simulink model "Torque_Vectoring_Controller_dSpace_RTI1401"  (R2016a)
settings: Solver=ode1  StartTime=0.0  StopTime=Inf  FixedStep=car.dt  RelTol=1e-3
PostLoadFcn:
  | , if any(exist('dsrtsu_mdlpostloadfcn', 'file') == [2, 3, 6]), try dsrtsu_mdlpostloadfcn('Execute', bdroot); catch fprintf('Error in PostLoadFcn (dsrtsu_mdlpostloadfcn) for model "%s":\n %s\n', bdroot, lasterr); end, end,
InitFcn:
  | clear_close
  | dataCar
  | optParam
  | structSensors
  | structSettings
  | structEstimPar
  | structAero
  | structVariables
  | readFuzzyFile
StartFcn:
  | clear_close
  | dataCar
  | optParam
  | structSensors
  | structSettings
  | structEstimPar
  | structAero
  | structVariables
  | readFuzzyFile
undefined symbols (not defined in the file or in its folder): car, optPar
libraries: fuzblock x1
(part 1 of 2)
PreSaveFcn:
  | , if any(exist('dsmpb_private', 'file') == [2, 3, 6]), try, dsmpb_private('dsmpb_mdlclblib', 'PreSave', bdroot); catch, disp(lasterr); end, end,
CloseFcn:
  | , if any(exist('dsmpb_private', 'file') == [2, 3, 6]), try, dsmpb_private('dsmpb_mdlclblib', 'Close', bdroot); catch, disp(lasterr); end, end,
settings Model: DSRTSU_INTERNAL_RTI_VER=490  DSRTSU_INTERNAL_RTI_TYPE=rti1401  DSRTSU_INTERNAL_RTIFPGA=80  DSMPB_DATASERVER_ModelPortLibVersion1=8  DSMPB_DATASERVER_DataServerVersion1=6  DSMPB_DATASERVER_DataServerStreamVersion1=3  Creator=Boon  LastModifiedBy=Boon
settings OptimizationCC: BlockReduction=off  OptimizeBlockIOStorage=off  BufferReuse=off  GlobalBufferReuse=off  ExpressionFolding=off  LocalBlockOutputs=off
settings HardwareCC: ProdBitPerPointer=32  ProdLargestAtomicInteger=Integer  ProdEndianess=BigEndian  ProdWordSize=32  ProdHWDeviceType=Custom Processor->Custom  TargetIntDivRoundTo=Zero  TargetEndianess=BigEndian  TargetHWDeviceType=Custom Processor->Custom
settings RTWCC: SystemTargetFile=rti1401.tlc  MakeCommand=make_rti  TemplateMakefile=rti1401.tmf  Description=dSPACE DS1401 Hardware Platform
settings STFCustomTargetCC: ParMdlRefBuildCompliant=on  GRTInterface=off  SystemTargetFile=rti1401.tlc
settings GRTTargetCC: CompOptLevelCompliant=off  ConcurrentExecutionCompliant=off  GeneratePreprocessorConditionals=Use local settings  CombineOutputUpdateFcns=off  MatFileLogging=off  CPPClassGenCompliant=off  UseToolchainInfoCompliant=off

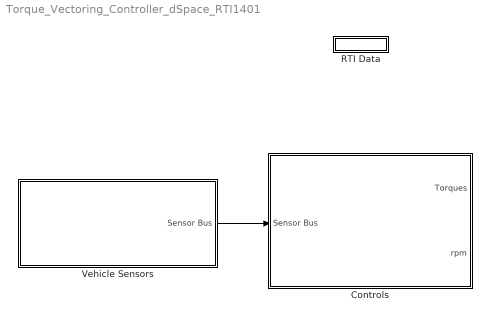
== system Torque_Vectoring_Controller_dSpace_RTI1401 ==
  Controls : Subsystem
  RTI Data : Subsystem  Tag=struct('RTIDataServer',struct('RTIDataServerVs','2','RTIModelDescription','struct(''main'',''Torque_Vectoring_Controller_dSpace_RTI1401'',''sub'','''',''isMp'',0)'))  LoadFcn="if exist('rtidc'), try,  rtidc('DataHostBlockClbLoad', gcbh); catch, disp(['Warning: ''LoadFcn'' for RTI Data block failed: ' lasterr]); end, end,"  mask(RTI_DATA_HOST){}
      mask help:
      | RTI Data Block.
      | This block is used by RTI to store internal model-dependent data.
      | Please keep this block on the root level of the model. Deleting this block will result in data loss.
      |
      | NEVER DELETE OR COPY THIS BLOCK!
      settings: CopyFcn="if exist('rtidc'), try,  rtidc('DataHostBlockClbCopy', gcbh); catch, disp(['Warning: ''CopyFcn'' for RTI Data block failed: ' lasterr]); end, end,"  DeleteFcn="if exist('rtidc'), try,  rtidc('DataHostBlockClbDelete', gcbh); catch, disp(['Warning: ''DeleteFcn'' for RTI Data block failed: ' lasterr]); end, end,"  ModelCloseFcn="if exist('rtidc'), try,  rtidc('DataHostBlockClbModelClose', gcbh); catch, disp(['Warning: ''ModelCloseFcn'' for RTI Data block failed: ' lasterr]); end, end,"  PreSaveFcn="if exist('rtidc'), try,  rtidc('DataHostBlockClbPreSave', gcbh); catch, disp(['Warning: ''PreSaveFcn'' for RTI Data block failed: ' lasterr]); end, end,"  PostSaveFcn="if exist('rtidc'), try,  rtidc('DataHostBlockClbPostSave', gcbh); catch, disp(['Warning: ''PostSaveFcn'' for RTI Data block failed: ' lasterr]); end, end,"  NameChangeFcn="if exist('rtidc'), try,  rtidc('DataHostBlockClbNameChange', gcbh); catch, disp(['Warning: ''NameChangeFcn'' for RTI Data block failed: ' lasterr]); end, end,"
      mask Help:
      | RTI Data Block.
      | This block is used by RTI to store internal model-dependent data.
      | Please keep this block on the root level of the model. Deleting this block will result in data loss.
      | 
      | NEVER DELETE OR COPY THIS BLOCK!
      mask Display:
      | text(0.5, 0.5, 'RTI Data', 'HorizontalAlignment', 'center');
      | plot([1 0]);
  Vehicle Sensors : Subsystem
  wires:
  Vehicle Sensors/1(" Sensor Bus") -> Controls/1(Sensor Bus)

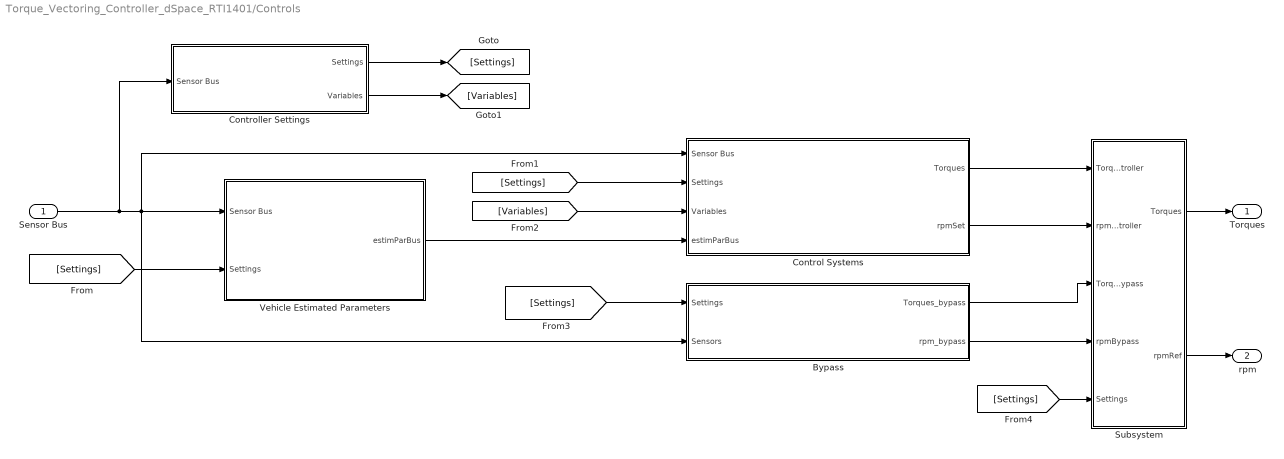
== system Torque_Vectoring_Controller_dSpace_RTI1401/Controls ==
  Sensor Bus : Inport
  Bypass : Subsystem
  Control Systems : Subsystem
  Controller Settings : Subsystem
  Subsystem : Subsystem
  Vehicle Estimated Parameters : Subsystem
  Torques : Outport
  rpm : Outport  Port=2
  wires:
  Sensor Bus/1 -> Controller Settings/1(Sensor Bus), Bypass/2(Sensors), Control Systems/1(Sensor Bus), Vehicle Estimated Parameters/1(Sensor Bus)
  [Settings] -> Vehicle Estimated Parameters/2(Settings)
  Vehicle Estimated Parameters/1(" estimParBus") -> Control Systems/4(estimParBus)
  Controller Settings/1(Settings) -> [Settings]
  [Settings] -> Control Systems/2(Settings)
  Controller Settings/2(Variables) -> [Variables]
  [Variables] -> Control Systems/3("Variables ")
  [Settings] -> Bypass/1(Settings)
  Control Systems/1(Torques) -> Subsystem/1(TorqueController)
  Subsystem/1(Torques) -> Torques/1
  Bypass/2(rpm_bypass) -> Subsystem/4(rpmBypass)
  Bypass/1(Torques_bypass) -> Subsystem/3(TorqueBypass)
  [Settings] -> Subsystem/5(Settings)
  Control Systems/2(rpmSet) -> Subsystem/2(rpmController)
  Subsystem/2(rpmRef) -> rpm/1

== system Torque_Vectoring_Controller_dSpace_RTI1401/RTI Data ==
  RTI Data Store : Subsystem  Tag="struct('private',struct('version',struct('dsVer',uint32(2),'dsVerCreation',uint32(2),'RTI',struct('ver','7.7','type','RTI1401')),'access',struct('type','Model','isPerm',1,'created',['18-Apr-2017 22:43:45'],'modified',['26-Apr-2017 00:23:53'],'location','')),'public',struct('main',struct('data',[]),'sub',struct('name',{{'Torque_Vectoring_Controller_dSpace_RTI1401'}},'data',{{struct('TH',struct('thTaskInfo',struct('taskType',{'TIMER','HWINT','TMRINT','SWINT','GLINT'},'tasksNumOf',{1,0,0,0,0},'srcIds',{{'TIMERA'},{},{},{},{}},'taskNames',{{['Timer Task 1']},{},{},{},{}})),'th_tc',struct('dataType','TASK','taskGroupId','','taskGroupList',{{}},'taskSchedulingPolicy','FCFS','taskType','TIMER','blkh',-1,'srcId','TIMERA','srcSgnName',['Timer A interrupt'],'srcCpuName','','taskName',['Timer Task 1  [0.001] s'],'taskNameDisplayExt','','smplTime',0.001,'smplTimeOffs',0,'hasFixedPriority',0,'priority',1,'hasFixedOvc',0,'ovcType',1,'ovcMax',1),'tc_th',struct('dataType','TASK','taskGroupId','','taskGroupList',{{}},'taskSchedulingPolicy','FCFS','taskType','TIMER','blkh',-1,'srcId','TIMERA','srcSgnName',['Timer A interrupt'],'srcCpuName','','taskName',['Timer Task 1  [0.001] s'],'taskNameDisplayExt','','smplTime',0.001,'smplTimeOffs',0,'hasFixedPriority',0,'priority',1,'hasFixedOvc',0,'ovcType',1,'ovcMax',1))}})))"  mask(RTI_DATA_STORE){}
      mask help:
      | RTI Data Store Block. This block is used by RTI to store internal model dependent data. Deleting this block will result in data loss.
      |
      | NEVER DELETE, COPY, OR MODIFY THIS BLOCK!
      mask Help:
      | RTI Data Store Block. This block is used by RTI to store internal model dependent data. Deleting this block will result in data loss.
      | 
      | NEVER DELETE, COPY, OR MODIFY THIS BLOCK!
      mask Display: text(0.5, 0.5, ' ', 'HorizontalAlignment', 'center');

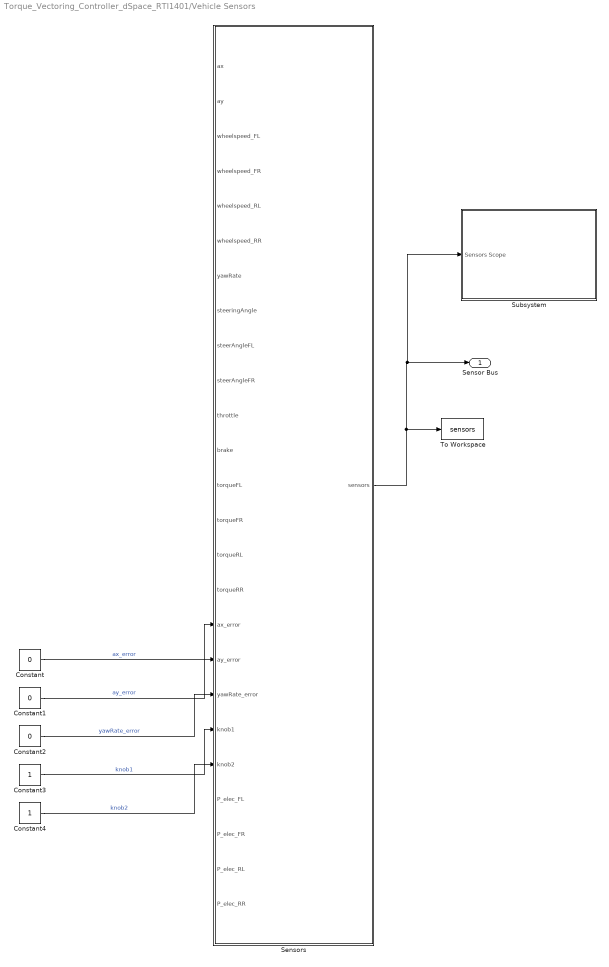
== system Torque_Vectoring_Controller_dSpace_RTI1401/Vehicle Sensors ==
  Constant : Constant  Value=0
  Constant1 : Constant  Value=0
  Constant2 : Constant  Value=0
  Constant3 : Constant
  Constant4 : Constant
  Sensors : MATLAB Function  TreatAsAtomicUnit=on
  Subsystem : Subsystem
      mask Display: image('Sensors Scope.png');
  To Workspace : ToWorkspace  VariableName=sensors  SaveFormat=Timeseries  SampleTime=-1
  " Sensor Bus" : Outport
  wires:
  Constant4/1 -> Sensors/21(knob2)  "knob2"
  Constant3/1 -> Sensors/20(knob1)  "knob1"
  Constant2/1 -> Sensors/19(yawRate_error)  "yawRate_error"
  Constant1/1 -> Sensors/18(ay_error)  "ay_error"
  Constant/1 -> Sensors/17(ax_error)  "ax_error"
  Sensors/1(sensors) -> Subsystem/1("Sensors Scope "), " Sensor Bus"/1, To Workspace/1

== system Torque_Vectoring_Controller_dSpace_RTI1401/Controls/Bypass ==
  Settings : Inport
  Sensors : Inport  Port=2
  MATLAB Function : MATLAB Function  TreatAsAtomicUnit=on
  Torques_bypass : Outport
  rpm_bypass : Outport  Port=2
  wires:
  Settings/1 -> MATLAB Function/1(settings)
  MATLAB Function/1(torqueBypass) -> Torques_bypass/1
  Sensors/1 -> MATLAB Function/2(sensors)
  MATLAB Function/2(rpmBypass) -> rpm_bypass/1

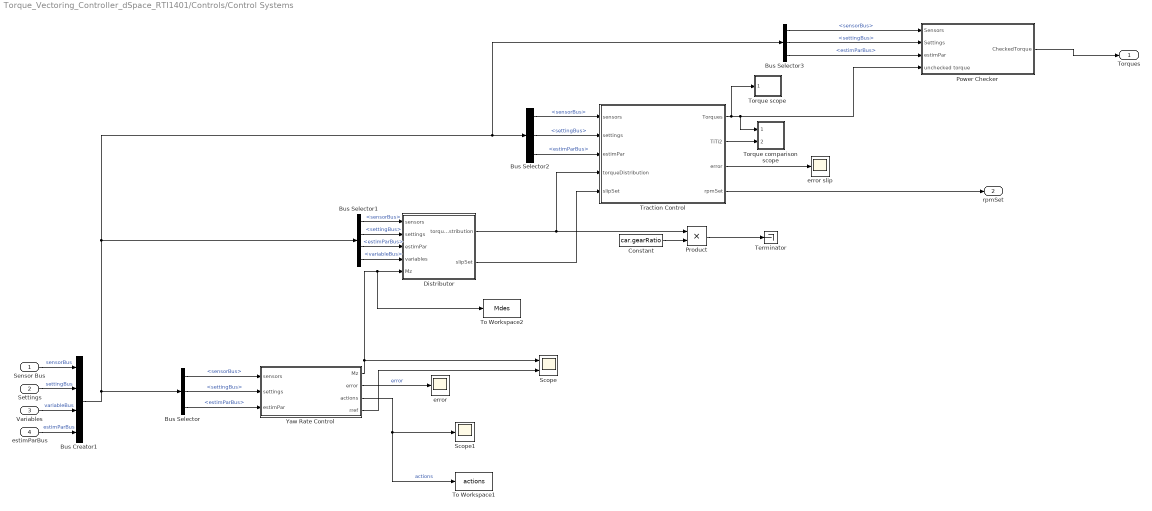
== system Torque_Vectoring_Controller_dSpace_RTI1401/Controls/Control Systems ==
  Sensor Bus : Inport
  Settings : Inport  Port=2
  "Variables " : Inport  Port=3
  estimParBus : Inport  Port=4
  Bus Creator1 : BusCreator  Inputs=4
  Bus Selector : BusSelector  OutputSignals=sensorBus,settingBus,estimParBus
  Bus Selector1 : BusSelector  OutputSignals=sensorBus,settingBus,estimParBus,variableBus
  Bus Selector2 : BusSelector  OutputSignals=sensorBus,settingBus,estimParBus
  Bus Selector3 : BusSelector  OutputSignals=sensorBus,settingBus,estimParBus
  Constant : Constant  Value=car.gearRatio
  Distributor : Subsystem
  Power Checker : Subsystem
  Product : Product
  Scope : Scope  NumInputPorts=2
  Scope1 : Scope
  Terminator : Terminator
  To Workspace1 : ToWorkspace  VariableName=actions  SaveFormat=Timeseries  SampleTime=-1
  To Workspace2 : ToWorkspace  VariableName=Mdes  SaveFormat=Timeseries  SampleTime=-1
  Torque comparison scope : Subsystem
  Torque scope : Subsystem
  Traction Control : MATLAB Function  TreatAsAtomicUnit=on
  Yaw Rate Control : MATLAB Function  TreatAsAtomicUnit=on
  error : Scope
  error slip : Scope
  Torques : Outport
  rpmSet : Outport  Port=2
  wires:
  Yaw Rate Control/1(Mz) -> To Workspace2/1, Distributor/5(Mz), Scope/1
  Settings/1 -> Bus Creator1/2  "settingBus"
  Sensor Bus/1 -> Bus Creator1/1  "sensorBus"
  Bus Selector/2 -> Yaw Rate Control/2(settings)  "<settingBus>"
  Bus Selector/1 -> Yaw Rate Control/1(sensors)  "<sensorBus>"
  Bus Selector1/3 -> Distributor/3(estimPar)  "<estimParBus>"
  Bus Selector1/2 -> Distributor/2(settings)  "<settingBus>"
  Bus Selector1/1 -> Distributor/1(sensors)  "<sensorBus>"
  Distributor/1(torqueDistribution) -> Product/1, Traction Control/4(torqueDistribution)
  Bus Selector2/3 -> Traction Control/3(estimPar)  "<estimParBus>"
  Bus Selector2/2 -> Traction Control/2(settings)  "<settingBus>"
  Bus Selector2/1 -> Traction Control/1(sensors)  "<sensorBus>"
  Bus Selector/3 -> Yaw Rate Control/3(estimPar)  "<estimParBus>"
  Distributor/2(slipSet) -> Traction Control/5(slipSet)
  Yaw Rate Control/2(error) -> error/1  "error"
  Yaw Rate Control/3(actions) -> To Workspace1/1, Scope1/1  "actions"
  estimParBus/1 -> Bus Creator1/4  "estimParBus"
  "Variables "/1 -> Bus Creator1/3  "variableBus"
  Bus Selector1/4 -> Distributor/4(variables)  "<variableBus>"
  Yaw Rate Control/4(rref) -> Scope/2
  Product/1 -> Terminator/1
  Constant/1 -> Product/2
  Bus Creator1/1 -> Bus Selector3/1, Bus Selector2/1, Bus Selector1/1, Bus Selector/1
  Traction Control/1(Torques) -> Torque scope/1(Torques), Torque comparison scope/1(Torques), Power Checker/4(unchecked torque)
  Traction Control/3(error) -> error slip/1
  Traction Control/4(rpmSet) -> rpmSet/1
  Traction Control/2(TiTi2) -> Torque comparison scope/2(Ti / Ti2)
  Bus Selector3/1 -> Power Checker/1(Sensors)  "<sensorBus>"
  Bus Selector3/2 -> Power Checker/2(Settings)  "<settingBus>"
  Power Checker/1(CheckedTorque) -> Torques/1
  Bus Selector3/3 -> Power Checker/3("estimPar  ")  "<estimParBus>"

== system Torque_Vectoring_Controller_dSpace_RTI1401/Controls/Controller Settings ==
  Sensor Bus : Inport
  Controller Settings : MATLAB Function  TreatAsAtomicUnit=on
  To Workspace : ToWorkspace  VariableName=settingOut  SaveFormat=Timeseries  SampleTime=-1
  Settings : Outport
  Variables : Outport  Port=2
  wires:
  Sensor Bus/1 -> Controller Settings/1(sensors)
  Controller Settings/2(variables) -> Variables/1
  Controller Settings/1(settings) -> To Workspace/1, Settings/1

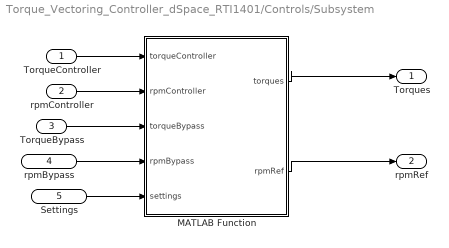
== system Torque_Vectoring_Controller_dSpace_RTI1401/Controls/Subsystem ==
  TorqueController : Inport
  rpmController : Inport  Port=2
  TorqueBypass : Inport  Port=3
  rpmBypass : Inport  Port=4
  Settings : Inport  Port=5
  MATLAB Function : MATLAB Function  TreatAsAtomicUnit=on
  Torques : Outport
  rpmRef : Outport  Port=2
  wires:
  MATLAB Function/1(torques) -> Torques/1
  TorqueController/1 -> MATLAB Function/1(torqueController)
  rpmController/1 -> MATLAB Function/2(rpmController)
  TorqueBypass/1 -> MATLAB Function/3(torqueBypass)
  rpmBypass/1 -> MATLAB Function/4(rpmBypass)
  MATLAB Function/2(rpmRef) -> rpmRef/1
  Settings/1 -> MATLAB Function/5(settings)

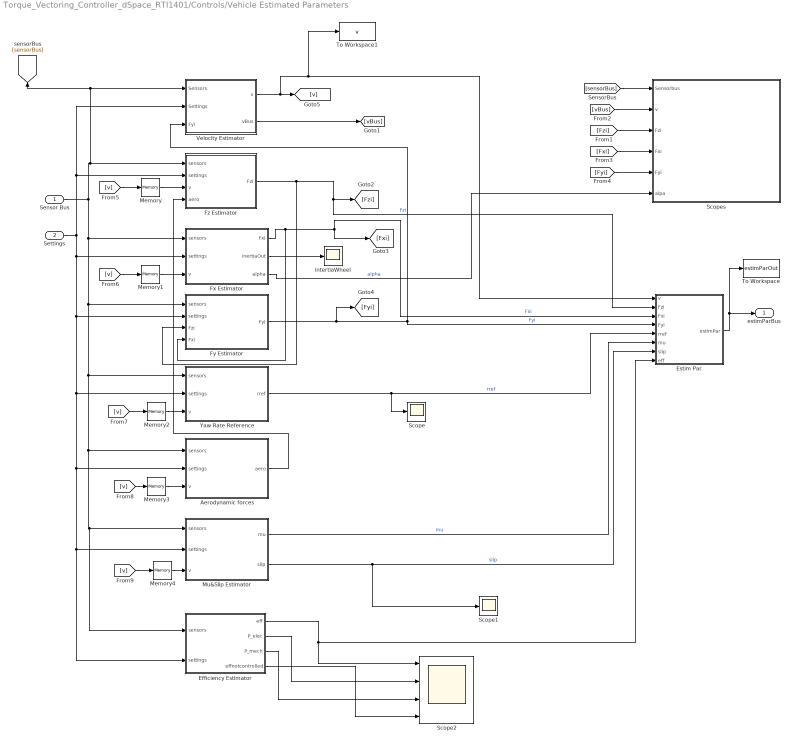
== system Torque_Vectoring_Controller_dSpace_RTI1401/Controls/Vehicle Estimated Parameters ==
  Sensor Bus : Inport
  Settings : Inport  Port=2
  Aerodynamic forces : MATLAB Function  TreatAsAtomicUnit=on
  Efficiency Estimator : MATLAB Function  TreatAsAtomicUnit=on
  Estim Par : MATLAB Function  TreatAsAtomicUnit=on
  "Fx Estimator " : MATLAB Function  TreatAsAtomicUnit=on
  "Fy Estimator " : MATLAB Function  TreatAsAtomicUnit=on
  "Fz Estimator " : MATLAB Function  TreatAsAtomicUnit=on
  Memory{,1..4} (5 alike) : Memory
  Mu&Slip Estimator : MATLAB Function  TreatAsAtomicUnit=on
  Scope : Scope
  Scope1 : Scope
  Scope2 : Scope  NumInputPorts=4
  Scopes : Subsystem
      mask Display: image('estimator.png');
  To Workspace : ToWorkspace  VariableName=estimParOut  SaveFormat=Timeseries  SampleTime=-1
  To Workspace1 : ToWorkspace  VariableName=v  SaveFormat=Timeseries  SampleTime=-1
  Velocity Estimator : Subsystem
  Yaw Rate Reference : MATLAB Function  TreatAsAtomicUnit=on
  intertiaWheel : Scope
  " estimParBus" : Outport
  wires:
  "Fx Estimator "/1(Fxi) -> Estim Par/3(Fxi), [Fxi], "Fy Estimator "/4(Fxi)  "Fxi"
  "Fz Estimator "/1(Fzi) -> "Fy Estimator "/3(Fzi), [Fzi], Estim Par/2(Fzi)  "Fzi"
  Yaw Rate Reference/1(rref) -> Estim Par/5(rref), Scope/1  "rref"
  "Fy Estimator "/1(Fyi) -> [Fyi], Velocity Estimator/3(Fyi), Estim Par/4(Fyi)  "Fyi"
  Estim Par/1(estimPar) -> To Workspace/1, " estimParBus"/1
  [vBus] -> Scopes/2(v)
  [Fzi] -> Scopes/3(Fzi)
  [sensorBus] -> Scopes/1(Sensorbus)
  [Fxi] -> Scopes/4(Fxi)
  Sensor Bus/1 -> "Fx Estimator "/1(sensors), Efficiency Estimator/1(sensors), Mu&Slip Estimator/1(sensors), Aerodynamic forces/1(sensors), Yaw Rate Reference/1(sensors), "Fy Estimator "/1(sensors), "Fz Estimator "/1(sensors), Velocity Estimator/1(Sensors), [sensorBus]
  Settings/1 -> Velocity Estimator/2(Settings), "Fz Estimator "/2(settings), Efficiency Estimator/2(settings), Mu&Slip Estimator/2(settings), Aerodynamic forces/2(settings), Yaw Rate Reference/2(settings), "Fy Estimator "/2(settings), "Fx Estimator "/2(settings)
  [Fyi] -> Scopes/5(Fyi)
  Velocity Estimator/1(v) -> Estim Par/1(v), To Workspace1/1, [v]
  Velocity Estimator/2(vBus) -> [vBus]
  Aerodynamic forces/1(aero) -> "Fz Estimator "/4(aero)
  Mu&Slip Estimator/1(mu) -> Estim Par/6(mu)  "mu"
  Mu&Slip Estimator/2(slip) -> Scope1/1, Estim Par/7(slip)  "slip"
  [v] -> Memory/1
  [v] -> Memory1/1
  [v] -> Memory2/1
  [v] -> Memory3/1
  [v] -> Memory4/1
  "Fx Estimator "/2(inertiaOut) -> intertiaWheel/1
  "Fx Estimator "/3(alpha) -> Scopes/6(alpa)  "alpha"
  Memory/1 -> "Fz Estimator "/3(v)
  Memory1/1 -> "Fx Estimator "/3(v)
  Memory2/1 -> Yaw Rate Reference/3(v)
  Memory3/1 -> Aerodynamic forces/3(v)
  Memory4/1 -> Mu&Slip Estimator/3(v)
  Efficiency Estimator/1(eff) -> Scope2/1, Estim Par/8(eff)
  Efficiency Estimator/2(P_elec) -> Scope2/2
  Efficiency Estimator/3(P_mech) -> Scope2/3
  Efficiency Estimator/4(effnotcontrolled) -> Scope2/4

== system Torque_Vectoring_Controller_dSpace_RTI1401/RTI Data/RTI Data Store ==
  RTI Data Store : Subsystem  mask(RTI_DATA_STORE){}
      mask help:
      | RTI Data Store Block. This block is used by RTI to store internal model dependent data. Deleting this block will result in data loss.
      |
      | NEVER DELETE, COPY, OR MODIFY THIS BLOCK!
      mask Help:
      | RTI Data Store Block. This block is used by RTI to store internal model dependent data. Deleting this block will result in data loss.
      | 
      | NEVER DELETE, COPY, OR MODIFY THIS BLOCK!
      mask Display: text(0.5, 0.5, ' ', 'HorizontalAlignment', 'center');

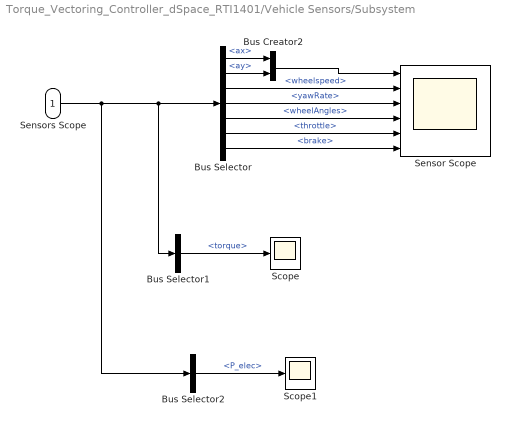
== system Torque_Vectoring_Controller_dSpace_RTI1401/Vehicle Sensors/Subsystem ==
  "Sensors Scope " : Inport
  Bus Creator2 : BusCreator  Inputs=2
  Bus Selector : BusSelector  OutputSignals=ax,ay,wheelspeed,yawRate,wheelAngles,throttle,brake
  Bus Selector1 : BusSelector  OutputSignals=torque
  Bus Selector2 : BusSelector  OutputSignals=P_elec
  Scope : Scope
  Scope1 : Scope
  Sensor Scope : Scope  NumInputPorts=6
  wires:
  Bus Selector/2 -> Bus Creator2/2  "<ay>"
  Bus Selector/4 -> Sensor Scope/3  "<yawRate>"
  Bus Selector/1 -> Bus Creator2/1  "<ax>"
  Bus Selector/6 -> Sensor Scope/5  "<throttle>"
  Bus Selector/7 -> Sensor Scope/6  "<brake>"
  Bus Selector/3 -> Sensor Scope/2  "<wheelspeed>"
  Bus Creator2/1 -> Sensor Scope/1
  "Sensors Scope "/1 -> Bus Selector2/1, Bus Selector1/1, Bus Selector/1
  Bus Selector/5 -> Sensor Scope/4  "<wheelAngles>"
  Bus Selector1/1 -> Scope/1  "<torque>"
  Bus Selector2/1 -> Scope1/1  "<P_elec>"

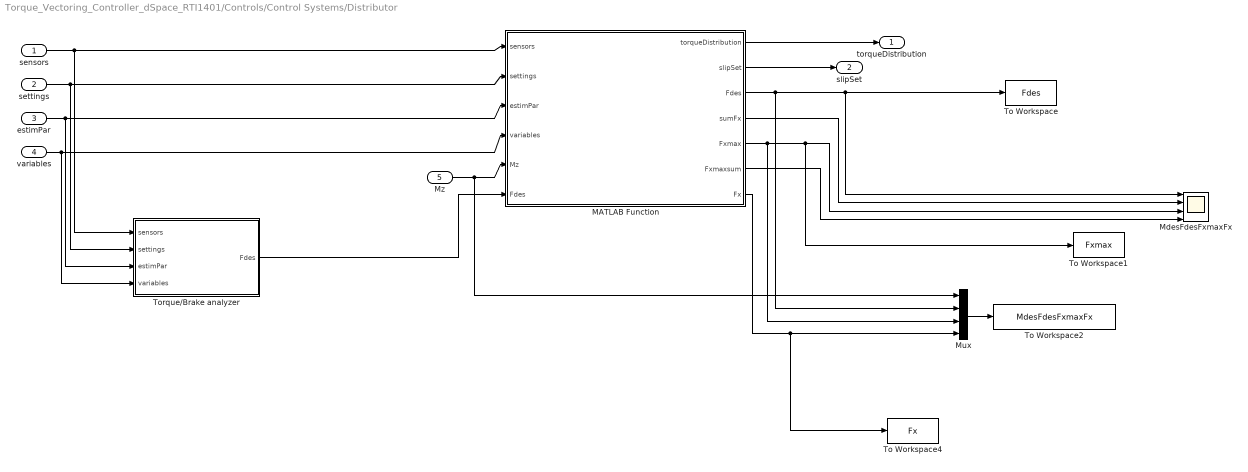
== system Torque_Vectoring_Controller_dSpace_RTI1401/Controls/Control Systems/Distributor ==
  sensors : Inport
  settings : Inport  Port=2
  estimPar : Inport  Port=3
  variables : Inport  Port=4
  Mz : Inport  Port=5
  MATLAB Function : MATLAB Function  TreatAsAtomicUnit=on
  MdesFdesFxmaxFx : Scope  NumInputPorts=4
  Mux : Mux
  To Workspace : ToWorkspace  VariableName=Fdes  SaveFormat=Timeseries  SampleTime=-1
  To Workspace1 : ToWorkspace  VariableName=Fxmax  SaveFormat=Timeseries  SampleTime=-1
  To Workspace2 : ToWorkspace  VariableName=MdesFdesFxmaxFx  SaveFormat=Timeseries  SampleTime=-1
  To Workspace4 : ToWorkspace  VariableName=Fx  SaveFormat=Timeseries  SampleTime=-1
  Torque/Brake analyzer : Subsystem
  torqueDistribution : Outport
  slipSet : Outport  Port=2
  wires:
  MATLAB Function/1(torqueDistribution) -> torqueDistribution/1
  sensors/1 -> Torque/Brake analyzer/1(sensors), MATLAB Function/1(sensors)
  settings/1 -> Torque/Brake analyzer/2(settings), MATLAB Function/2(settings)
  estimPar/1 -> Torque/Brake analyzer/3(estimPar), MATLAB Function/3(estimPar)
  Mz/1 -> Mux/1, MATLAB Function/5(Mz)
  MATLAB Function/2(slipSet) -> slipSet/1
  variables/1 -> Torque/Brake analyzer/4(variables), MATLAB Function/4(variables)
  MATLAB Function/3(Fdes) -> Mux/2, MdesFdesFxmaxFx/1, To Workspace/1
  MATLAB Function/4(sumFx) -> MdesFdesFxmaxFx/2
  MATLAB Function/6(Fxmaxsum) -> MdesFdesFxmaxFx/4
  Mux/1 -> To Workspace2/1
  MATLAB Function/7(Fx) -> To Workspace4/1, Mux/4
  MATLAB Function/5(Fxmax) -> To Workspace1/1, MdesFdesFxmaxFx/3, Mux/3
  Torque/Brake analyzer/1(Fdes) -> MATLAB Function/6("Fdes ")

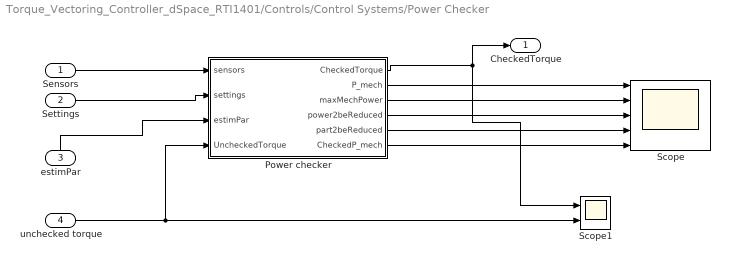
== system Torque_Vectoring_Controller_dSpace_RTI1401/Controls/Control Systems/Power Checker ==
  Sensors : Inport
  Settings : Inport  Port=2
  "estimPar  " : Inport  Port=3
  unchecked torque : Inport  Port=4
  Power checker : MATLAB Function  TreatAsAtomicUnit=on
  Scope : Scope  NumInputPorts=5
  Scope1 : Scope  NumInputPorts=2
  CheckedTorque : Outport
  wires:
  Sensors/1 -> Power checker/1(sensors)
  Settings/1 -> Power checker/2(settings)
  Power checker/1(CheckedTorque) -> Scope1/1, CheckedTorque/1
  "estimPar  "/1 -> Power checker/3(estimPar)
  unchecked torque/1 -> Scope1/2, Power checker/4(UncheckedTorque)
  Power checker/2(P_mech) -> Scope/1
  Power checker/3(maxMechPower) -> Scope/2
  Power checker/4(power2beReduced) -> Scope/3
  Power checker/5(part2beReduced) -> Scope/4
  Power checker/6(CheckedP_mech) -> Scope/5

== system Torque_Vectoring_Controller_dSpace_RTI1401/Controls/Control Systems/Torque comparison scope ==
  Torques : Inport
  Ti / Ti2 : Inport  Port=2
  Demux : Demux  Outputs=2
  Scope2 : Scope  NumInputPorts=3
  wires:
  Torques/1 -> Scope2/1
  Demux/1 -> Scope2/2  "Ti"
  Demux/2 -> Scope2/3  "Ti2"
  Ti / Ti2/1 -> Demux/1

== system Torque_Vectoring_Controller_dSpace_RTI1401/Controls/Control Systems/Torque scope ==
  Torques : Inport
  Constant2 : Constant  Value=car.gearRatio
  Product2 : Product
  To Workspace : ToWorkspace  VariableName=torques  SaveFormat=Timeseries  SampleTime=-1
  Torques scope : Scope
  wires:
  Torques/1 -> Product2/1
  Constant2/1 -> Product2/2
  Product2/1 -> To Workspace/1, Torques scope/1

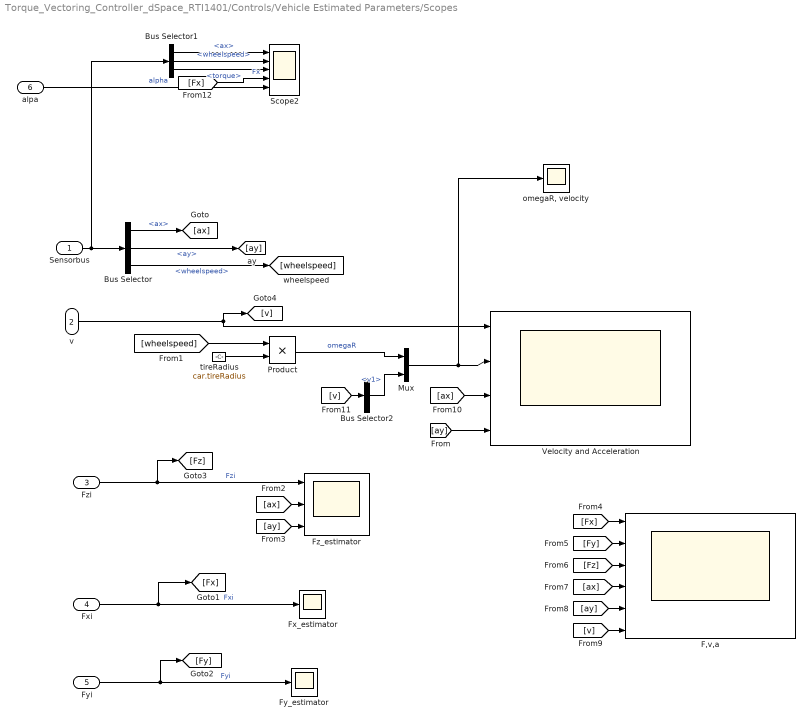
== system Torque_Vectoring_Controller_dSpace_RTI1401/Controls/Vehicle Estimated Parameters/Scopes ==
  Sensorbus : Inport
  v : Inport  Port=2
  Fzi : Inport  Port=3
  Fxi : Inport  Port=4
  Fyi : Inport  Port=5
  alpa : Inport  Port=6
  Bus Selector : BusSelector  OutputSignals=ax,ay,wheelspeed
  Bus Selector1 : BusSelector  OutputSignals=ax,wheelspeed,torque
  Bus Selector2 : BusSelector  OutputSignals=v1
  F,v,a : Scope  NumInputPorts=6
  Fx_estimator : Scope
  Fy_estimator : Scope
  Fz_estimator : Scope  NumInputPorts=3
  Mux : Mux  Inputs=2
  Product : Product
  Scope2 : Scope  NumInputPorts=5
  "Velocity and Acceleration " : Scope  NumInputPorts=4
  "omegaR, velocity" : Scope
  tireRadius : Constant  Value=car.tireRadius
  wires:
  tireRadius/1 -> Product/2
  Product/1 -> Mux/1  "omegaR"
  v/1 -> "Velocity and Acceleration "/1, [v]
  Fzi/1 -> [Fz], Fz_estimator/1  "Fzi"
  Sensorbus/1 -> Bus Selector1/1, Bus Selector/1
  Bus Selector/2 -> [ay]  "<ay>"
  [ay] -> "Velocity and Acceleration "/4
  Bus Selector/3 -> [wheelspeed]  "<wheelspeed>"
  [wheelspeed] -> Product/1
  Bus Selector/1 -> [ax]  "<ax>"
  [ax] -> Fz_estimator/2
  [ay] -> Fz_estimator/3
  Fxi/1 -> [Fx], Fx_estimator/1  "Fxi"
  Fyi/1 -> [Fy], Fy_estimator/1  "Fyi"
  [Fz] -> F,v,a/3
  [Fy] -> F,v,a/2
  [Fx] -> F,v,a/1
  [ax] -> F,v,a/4
  [ay] -> F,v,a/5
  [v] -> F,v,a/6
  [ax] -> "Velocity and Acceleration "/3
  [v] -> Bus Selector2/1
  Bus Selector2/1 -> Mux/2  "<v1>"
  Mux/1 -> "Velocity and Acceleration "/2, "omegaR, velocity"/1
  Bus Selector1/1 -> Scope2/1  "<ax>"
  Bus Selector1/2 -> Scope2/2  "<wheelspeed>"
  Bus Selector1/3 -> Scope2/3  "<torque>"
  [Fx] -> Scope2/4  "Fx"
  alpa/1 -> Scope2/5  "alpha"

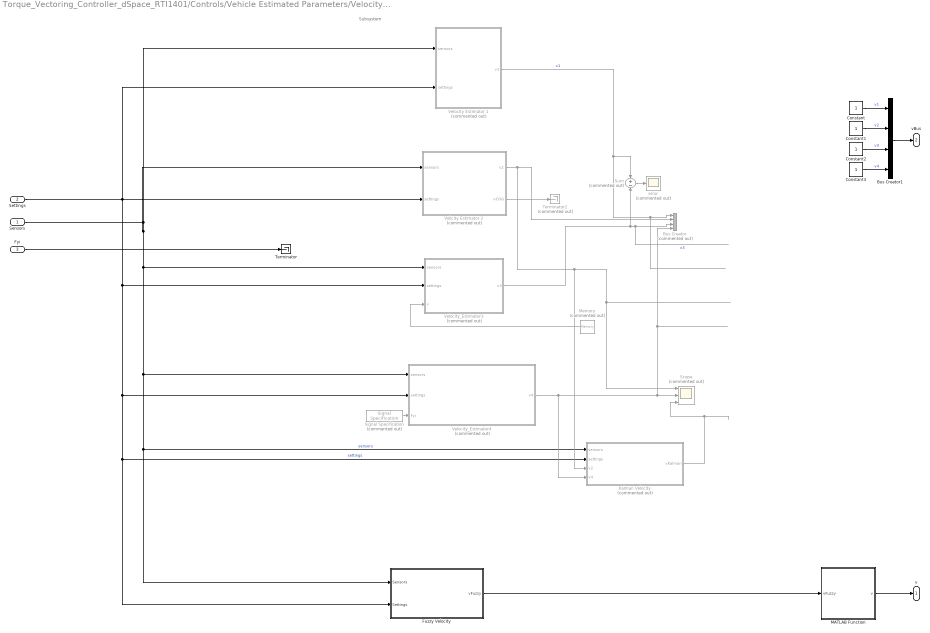
== system Torque_Vectoring_Controller_dSpace_RTI1401/Controls/Vehicle Estimated Parameters/Velocity Estimator ==
  note: Subsystem
  Sensors : Inport
  Settings : Inport  Port=2
  Fyi : Inport  Port=3
  Bus Creator : BusCreator  Commented=on  Inputs=4
  Bus Creator1 : BusCreator  Inputs=4
  Constant{,1..3} (4 alike) : Constant
  Fuzzy Velocity : Subsystem
  Kalman Velocity : MATLAB Function  Commented=on  TreatAsAtomicUnit=on
  MATLAB Function : MATLAB Function  TreatAsAtomicUnit=on
  Memory : Memory  Commented=on
  Scope : Scope  Commented=on  NumInputPorts=3
  Signal Specification : SignalSpecification  Commented=on  Dimensions=[4,1]
  Sum : Sum  Commented=on  Inputs=+-
  Terminator : Terminator
  Terminator2 : Terminator  Commented=on
  Velicity Estimator 2 : MATLAB Function  Commented=on  TreatAsAtomicUnit=on
  Velocity Estimator 1 : MATLAB Function  Commented=on  TreatAsAtomicUnit=on
  Velocity_Estimator3 : MATLAB Function  Commented=on  TreatAsAtomicUnit=on
  Velocity_Estimator4 : MATLAB Function  Commented=on  TreatAsAtomicUnit=on
  error : Scope  Commented=on
  v : Outport
  vBus : Outport  Port=2
  wires:
  Sensors/1 -> Velicity Estimator 2/1(sensors), Velocity_Estimator3/1(sensors), Kalman Velocity/1(sensors), Fuzzy Velocity/1(Sensors), Velocity_Estimator4/1(sensors), Velocity Estimator 1/1(sensors)  "sensors"
  Settings/1 -> Velocity_Estimator3/2(settings), Kalman Velocity/2(settings), Fuzzy Velocity/2(Settings), Velocity_Estimator4/2(settings), Velicity Estimator 2/2(settings), Velocity Estimator 1/2(settings)  "settings"
  Fuzzy Velocity/1(vFuzzy) -> MATLAB Function/1(vFuzzy)
  Velicity Estimator 2/1(v2) -> Kalman Velocity/3(v2), Scope/1, Bus Creator/2
  Velocity_Estimator4/1(v4) -> Kalman Velocity/4(v4), Bus Creator/4, Scope/2
  Kalman Velocity/1(vKalman) -> Scope/3
  MATLAB Function/1(v) -> v/1
  Signal Specification/1 -> Velocity_Estimator4/3(Fyi)
  Velocity_Estimator3/1(v3) -> Bus Creator/3, Sum/2  "v3"
  Velocity Estimator 1/1(v1) -> Sum/1, Bus Creator/1  "v1"
  Velicity Estimator 2/2(vCOG) -> Terminator2/1
  Memory/1 -> Velocity_Estimator3/3(v)
  Sum/1 -> error/1
  Bus Creator1/1 -> vBus/1
  Constant/1 -> Bus Creator1/1  "v1"
  Constant2/1 -> Bus Creator1/3  "v3"
  Constant1/1 -> Bus Creator1/2  "v2"
  Constant3/1 -> Bus Creator1/4  "v4"
  Fyi/1 -> Terminator/1

== system Torque_Vectoring_Controller_dSpace_RTI1401/RTI Data/RTI Data Store/RTI Data Store ==
  RTI Data Store : Subsystem  mask(RTI_DATA_STORE){}
      mask help:
      | RTI Data Store Block. This block is used by RTI to store internal model dependent data. Deleting this block will result in data loss.
      |
      | NEVER DELETE, COPY, OR MODIFY THIS BLOCK!
      mask Help:
      | RTI Data Store Block. This block is used by RTI to store internal model dependent data. Deleting this block will result in data loss.
      | 
      | NEVER DELETE, COPY, OR MODIFY THIS BLOCK!
      mask Display: text(0.5, 0.5, ' ', 'HorizontalAlignment', 'center');

== system Torque_Vectoring_Controller_dSpace_RTI1401/Controls/Control Systems/Distributor/Torque//Brake analyzer ==
  sensors : Inport
  settings : Inport  Port=2
  estimPar : Inport  Port=3
  variables : Inport  Port=4
  MATLAB Function1 : MATLAB Function  TreatAsAtomicUnit=on
  Fdes : Outport
  wires:
  MATLAB Function1/1(Fdes) -> Fdes/1
  sensors/1 -> MATLAB Function1/1(sensors)
  settings/1 -> MATLAB Function1/2(settings)
  variables/1 -> MATLAB Function1/4(variables)
  estimPar/1 -> MATLAB Function1/3(estimPar)

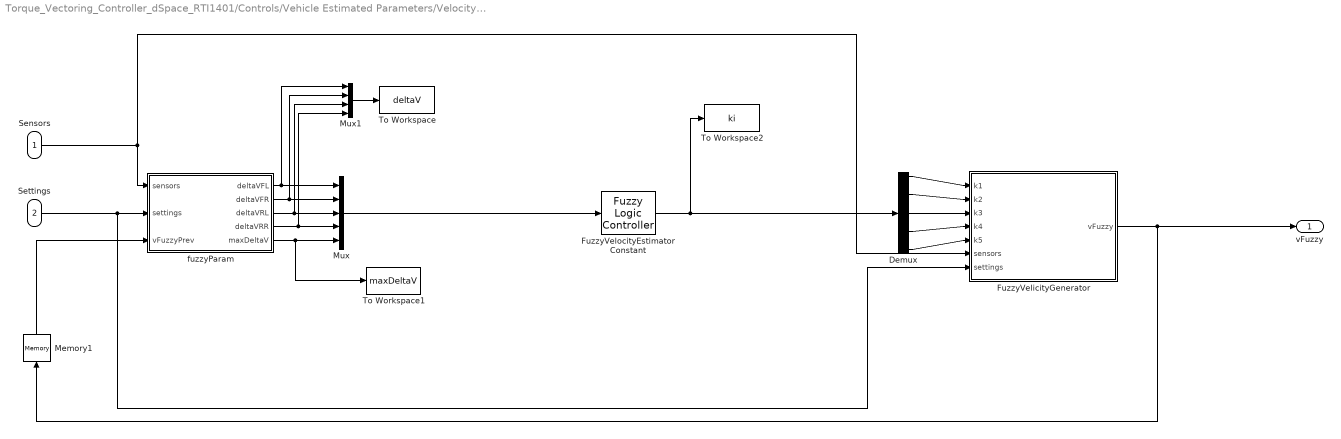
== system Torque_Vectoring_Controller_dSpace_RTI1401/Controls/Vehicle Estimated Parameters/Velocity Estimator/Fuzzy Velocity ==
  Sensors : Inport
  Settings : Inport  Port=2
  Demux : Demux  Outputs=5
  FuzzyVelicityGenerator : MATLAB Function  TreatAsAtomicUnit=on
  FuzzyVelocityEstimatorConstant : fuzblock/Fuzzy Logic  Controller  fis=fuzzyVelocityEstimatorConstant
  Memory1 : Memory
  Mux : Mux  Inputs=5
  Mux1 : Mux
  To Workspace : ToWorkspace  VariableName=deltaV  SaveFormat=Timeseries  SampleTime=-1
  To Workspace1 : ToWorkspace  VariableName=maxDeltaV  SaveFormat=Timeseries  SampleTime=-1
  To Workspace2 : ToWorkspace  VariableName=ki  SaveFormat=Timeseries  SampleTime=-1
  fuzzyParam : MATLAB Function  TreatAsAtomicUnit=on
  vFuzzy : Outport
  wires:
  fuzzyParam/4(deltaVRR) -> Mux1/4, Mux/4
  fuzzyParam/2(deltaVFR) -> Mux1/2, Mux/2
  fuzzyParam/3(deltaVRL) -> Mux1/3, Mux/3
  fuzzyParam/5(maxDeltaV) -> To Workspace1/1, Mux/5
  FuzzyVelicityGenerator/1(vFuzzy) -> vFuzzy/1, Memory1/1
  fuzzyParam/1(deltaVFL) -> Mux1/1, Mux/1
  Demux/5 -> FuzzyVelicityGenerator/5(k5)
  Memory1/1 -> fuzzyParam/3(vFuzzyPrev)
  Demux/1 -> FuzzyVelicityGenerator/1(k1)
  Demux/4 -> FuzzyVelicityGenerator/4(k4)
  Demux/3 -> FuzzyVelicityGenerator/3(k3)
  Sensors/1 -> FuzzyVelicityGenerator/6(sensors), fuzzyParam/1(sensors)
  Settings/1 -> fuzzyParam/2(settings), FuzzyVelicityGenerator/7(settings)
  Demux/2 -> FuzzyVelicityGenerator/2(k2)
  Mux/1 -> FuzzyVelocityEstimatorConstant/1
  FuzzyVelocityEstimatorConstant/1 -> To Workspace2/1, Demux/1
  Mux1/1 -> To Workspace/1

== system Torque_Vectoring_Controller_dSpace_RTI1401/RTI Data/RTI Data Store/RTI Data Store/RTI Data Store ==
  RTI Data Store : Subsystem  mask(RTI_DATA_STORE){}
      mask help:
      | RTI Data Store Block. This block is used by RTI to store internal model dependent data. Deleting this block will result in data loss.
      |
      | NEVER DELETE, COPY, OR MODIFY THIS BLOCK!
      mask Help:
      | RTI Data Store Block. This block is used by RTI to store internal model dependent data. Deleting this block will result in data loss.
      | 
      | NEVER DELETE, COPY, OR MODIFY THIS BLOCK!
      mask Display: text(0.5, 0.5, ' ', 'HorizontalAlignment', 'center');

== system Torque_Vectoring_Controller_dSpace_RTI1401/RTI Data/RTI Data Store/RTI Data Store/RTI Data Store/RTI Data Store ==

== matlab function Torque_Vectoring_Controller_dSpace_RTI1401/Controls/Control Systems/Traction Control ==
  data: sensors input; Torques output; settings input; estimPar input; torqueDistribution input; slipSet input; car parameter; TiTi2 output; error output; rpmSet output
function [Torques, TiTi2, error, rpmSet] = Traction(sensors, settings, estimPar, torqueDistribution, slipSet, car)

error =[0 0 0 0]';
persistent errorInt; if isempty(errorInt); errorInt=[0 0 0 0]'; end
persistent errorD; if isempty(errorD); errorD=[0 0 0 0]'; end
persistent errorPrev; if isempty(errorPrev); errorPrev=[0 0 0 0]'; end

%persistent wi_prev; if isempty(wi_prev); wi_prev=[0 0 0 0]'; end
%persistent SR_expected; if isempty(SR_expected); SR_expected=zeros(4, 8); end
%persistent wvi_prev; if isempty(wvi_prev); wvi_prev=[0 0 0 0]'; end

persistent TiPrev; if isempty(TiPrev); TiPrev=[0 0 0 0]'; end

persistent errorInt2; if isempty(errorInt2); errorInt2=[0 0 0 0]'; end
persistent Ti; if isempty(Ti); Ti=[0 0 0 0]'; end
persistent Ti2; if isempty(Ti2); Ti2=[0 0 0 0]'; end

rpmSet = [20000;20000;20000;20000];

if settings.TC == 1

    slipRatioTarget = slipSet;
    dist = estimPar.Fzi/sum(estimPar.Fzi);
    
    Kp = 100*dist*10;
    Ki = 40*dist*1000;
    Kd = 0*dist/100;
    Kv = 70/100;
    Mu = 1,40;
    
    Kp2 = 20*dist/1000;
    Ki2 = 40*dist/1000;
    
    %normal non linear torque control
    error = slipRatioTarget - estimPar.slip;
    
    errorInt = errorInt + error*car.dt;
    errorInt = min(max(errorInt,-0.001*[1;1;1;1]),0.003*[1;1;1;1]);
    errorD = min(max(errorD*0.1 + 0.9*(error - errorPrev)/car.dt,-25),25);
    lambdaD = Kp.*error + Ki.*errorInt + Kd.*errorD;
    Ti = lambdaD*car.tireInertia*max(estimPar.v,0)^Kv/car.tireRadius + sign(torqueDistribution).*estimPar.Fzi*(Mu)*car.tireRadius;
    Ti = Ti / car.gearRatio;
    
    %optimum seeking
    dFds = dFdsCalculator(estimPar.Fxi,estimPar.slip);
    error2 = dFds - 0;
    errorInt2 = errorInt2 + error2*car.dt;
    errorInt2 = min(max(errorInt2,-500*[1;1;1;1]),500*[1;1;1;1]);
    lambdaD2 = Kp2.*error2 + Ki2.*errorInt2;
    Ti2 = lambdaD2*car.tireInertia*max(estimPar.v,0)^Kv/car.tireRadius + sign(torqueDistribution).*estimPar.Fzi*(car.TC_mu)*car.tireRadius;
    Ti2 = Ti2 / car.gearRatio;
    
    for i=1:4
        if abs(error(i)) < 0.05
            Ti(i) = Ti2(i);
        end
    end
    
    if estimPar.v < 1/3.6
        %Ti = [80 80 180 180]';
        errorInt = [0 0 0 0]';
    end

    if sensors.throttle < 0.1
        errorInt = [0 0 0 0]';
    end
    
    lowerBoundary = TiPrev - 100/car.gearRatio;
    upperBoundary = TiPrev + 100/car.gearRatio;

    Ti = min(max(Ti,lowerBoundary),upperBoundary);
    
    TiPrev = Ti;
    errorPrev = error;
    
    Torques = Ti;
    for i=1:4
        if torqueDistribution(i) > 0
            Torques(i) = max(min(Torques(i),torqueDistribution(i)),0); 
        else
            Torques(i) = min(max(Torques(i),torqueDistribution(i)),0);
        end
    end
    
    
else
    Torques = torqueDistribution;
end

checkTorquemax = find((Torques > car.motor.Tmax)==1); %Limit torques to max torque
Torques(checkTorquemax)=car.motor.Tmax(checkTorquemax);



%wi_prev = sensors.wheelspeed;
%wvi_prev = sensors.wheelspeedi;

TiTi2 = [Ti;Ti2];

end

function [dFds] = dFdsCalculator(Fx,slipRatio)
N = 6;

persistent slipVector, if isempty(slipVector); slipVector = zeros(N,4); end
persistent FxVector, if isempty(FxVector); FxVector = zeros(N,4); end


FxVector(1,:) = Fx;
slipVector(1,:) = slipRatio;

dFds = [0;0;0;0];

for i=1:4
    p1 = polyfit(slipVector(:,i),FxVector(:,i),1);
    p2 = polyfit(FxVector(:,i),slipVector(:,i),1);
    
    rico1 = p1(1);
    rico2 = 1/p2(1);
    
    rico = sign(min(abs(rico1),abs(rico2)))*min(abs(rico1),abs(rico2));

    dFds(i) = max(min(rico,20000),-20000);
end

% shift list one
dummy = FxVector(1:N-1,:);
FxVector = [[0,0,0,0];dummy];
dummy = slipVector(1:N-1,:);
slipVector = [[0,0,0,0];dummy];

end

== matlab function Torque_Vectoring_Controller_dSpace_RTI1401/Controls/Vehicle Estimated Parameters/Mu&Slip Estimator ==
  data: sensors input; mu output; settings input; slip output; v input; car parameter
function [mu,slip]= mu_slip(sensors, settings,v,car)
if isempty(v); v =0;end
yawRate = [0;0;sensors.yawRate];
dist = [car.lf car.lf -car.lr -car.lr;
    car.tw/2 -car.tw/2 car.tw/2 -car.tw/2;
    0 0 0 0];
wheelAngle = (sensors.wheelAngles(1)+sensors.wheelAngles(2))/2;

mu=[car.mu;car.mu;car.mu;car.mu];

omegaR = sensors.wheelspeed*car.tireRadius;
vWheel=zeros(4,1);
vWheel_m=zeros(3,4);

for i=1:4;
    v_sleep=cross(yawRate,dist(:,i));
    vWheel_m(:,i) = [v;0;0] + v_sleep;
    vWheel(i,1) = sqrt(vWheel_m(1,i)^2+vWheel_m(2,i)^2);
end

%state.slipRatio = (sensor.omegaiWheel * car.wheelRadius - wvi)./max((sensor.omegaiWheel * car.wheelRadius),1);

if sensors.ax > 0
    slip = (omegaR - vWheel)./omegaR;
elseif sensors.ax < 0
    slip = (omegaR - vWheel)./vWheel;
else
    slip = [0;0;0;0];
end
end

== matlab function Torque_Vectoring_Controller_dSpace_RTI1401/Controls/Control Systems/Yaw Rate Control ==
  data: sensors input; Mz output; settings input; estimPar input; car parameter; error output; actions output; rref output
function [Mz,error,actions,rref]= yawRateControl(sensors, settings, estimPar, car)
%Function that controls the moment around the z-axis
%INPUTS:
%OUTPUT: Moment of the car around Z-axis [Nm]

Mz = 0;
Mz_temp = 0;
rref = estimPar.rref;
error = 0;


wheelAngle = (sensors.wheelAngles(1)+sensors.wheelAngles(2))/2;

%For analyzation
P_Action = 0;
I_Action = 0;
D_Action = 0;

steeringWheel_Action = 0;
yawRate_Action = 0;

persistent Mz_memory; if isempty(Mz_memory); Mz_memory = 0; end
persistent errorInt; if isempty(errorInt); errorInt = 0; end
persistent errorDev; if isempty(errorDev); errorDev = 0; end
persistent prevError; if isempty(prevError); prevError = 0; end
persistent prevWheelAngle; if isempty(prevWheelAngle); prevWheelAngle = 0; end
persistent prevRref; if isempty(prevRref); prevRref = 0; end

%if settings.YRCMode == 1
error = estimPar.rref - sensors.yawRate;
errorInt = errorInt + error*car.dt;
errorInt = min(max(errorInt,-car.YRC.intLimit),car.YRC.intLimit);
errorDev = (error - prevError)/car.dt;
wheelAngleDev = (wheelAngle - prevWheelAngle)/car.dt;
rrefDev = (estimPar.rref - prevRref)/car.dt;

velocityGain = min(max(1 - (estimPar.v - car.YRC.changeVelocity)*car.YRC.slope,0),1);

Mz_temp = (car.YRC.Kp*error + car.YRC.Ki*errorInt + car.YRC.Kd*errorDev...
    +car.YRC.Ks*wheelAngleDev + car.YRC.Kr*rrefDev)*velocityGain;
Mz_temp = max(min(Mz_temp,car.YRC.maxValue),-car.YRC.maxValue);
Mz_memory=Mz_memory+Mz_temp;

P_Action = car.YRC.Kp*error;
I_Action = car.YRC.Ki*errorInt;
D_Action = car.YRC.Kd*errorDev;
steeringWheel_Action = car.YRC.Ks*wheelAngle;
yawRate_Action = car.YRC.Kr*estimPar.rref;

actions = [P_Action;I_Action;D_Action;steeringWheel_Action;yawRate_Action];
prevError = error;
prevWheelAngle = wheelAngle;
prevRref = estimPar.rref;
%end


% if settings.YRCMode == 2
%     error = estimPar.rref - sensors.yawRate;
%     integral = integral + error*car.dt;
%     derivative = (error - prevError)/car.dt;
%
%     Mz_temp = car.YRC.Kp*error + car.YRC.Ki*integral + car.YRC.Kd*derivative...
%         +car.YRC.Ks*wheelAngle + car.YRC.Kr*estimPar.rref;
%     Mz_temp = max(min(Mz_temp,car.YRC.maxValue),-car.YRC.maxValue);
%
%     prevError = error;
% end





%YRC enabled
if settings.YRC ==1
    Mz = Mz_memory;
    
    %YRC disabled
else
    Mz = 0;
end

if car.YRC.minV > estimPar.v
    Mz = 0; %if speed is too low, don't activate yaw rate control
    errorInt = 0;
    prevError = 0;
end



rref=estimPar.rref;

== matlab function Torque_Vectoring_Controller_dSpace_RTI1401/Controls/Controller Settings/Controller Settings ==
  data: settings output Bus: settingBus; sensors input; variables output Bus: variableBus
function [settings,variables] = settingController(sensors)

%% Settings
velocityEstimation_Temp = 1;
YRCMode_Temp = 1;
torqueMode_Temp = 0;
YRC_Temp = 0;
TC_Temp = 0;
unlimitedFx_Temp = 0;
effEstimation_Temp = 2;


%if sensors.knob1 == 1
    YRC_Temp = 1;
%end

%if sensors.knob1 == 1
    torqueMode_Temp = 2; %Change distributor mode
%end

%if sensors.knob2 == 1
    YRCMode_Temp = 1;
    TC_Temp = 0;
    unlimitedFx_Temp = 0;
    TV_bypass_Temp = 0;
%end

%if sensors.knob2 == 2
    %YRCMode_Temp = 2;
%end

%% Variables
TD_percentage_Temp = 1;


%% Declaration Settings

settings.velocityEstimation = velocityEstimation_Temp;
settings.torqueMode = torqueMode_Temp;
settings.YRC = YRC_Temp;
settings.YRCMode = YRCMode_Temp;
settings.distributorMode = 0;

settings.Fsens = 50; %value between 0 and 100
% 100 --> Fdes is really important
% 0 --> Mdes is really important

settings.Fxsens = 1;

settings.TC = TC_Temp;
settings.unlimitedFx = unlimitedFx_Temp;
settings.TV_bypass = TV_bypass_Temp;
settings.effEstimation = effEstimation_Temp;

%% Declaration Variables
variables.TD_percentage = TD_percentage_Temp;

== matlab function Torque_Vectoring_Controller_dSpace_RTI1401/Controls/Vehicle Estimated Parameters/Fz Estimator  ==
  data: sensors input; Fzi output; settings input; v input; car parameter; aero input
function Fzi = Fz_Estimator(sensors, settings, v,car, aero)
if isempty(v); v =0;end
%Dynamical loads 
%Without taking suspension into account


FFA = car.g*car.mass*car.lr/car.wb - (car.h/car.wb)*(car.mass*sensors.ax) - aero.FD*((car.h+aero.lever_FD(2))/car.wb) - aero.FL*((car.lr-aero.lever_FL(1))/car.wb); %dyn load Front Axle
FRA = car.g*car.mass*car.lf/car.wb + (car.h/car.wb)*(car.mass*sensors.ax) + aero.FD*((car.h+aero.lever_FD(2))/car.wb) - aero.FL*((car.lf+aero.lever_FL(1))/car.wb); %dyn load Rear Axle


FFL = FFA/2 - (car.h/(2*car.tw))*(car.mass*sensors.ay);
FFR = FFA/2 + (car.h/(2*car.tw))*(car.mass*sensors.ay);
FRL = FRA/2 - (car.h/(2*car.tw))*(car.mass*sensors.ay);
FRR = FRA/2 + (car.h/(2*car.tw))*(car.mass*sensors.ay);


Fzi = [FFL;FFR;FRL;FRR];

== matlab function Torque_Vectoring_Controller_dSpace_RTI1401/Controls/Vehicle Estimated Parameters/Fx Estimator  ==
  data: sensors input; Fxi output; settings input; v input; car parameter; inertiaOut output; alpha output
function [Fxi,inertiaOut, alpha]= Fx_Estimator(sensors, settings, v, car)
%OPM: gearratio zit al verwerkt in sensors.torque (= wheelTorque)

persistent wheelspeedPrev; if isempty(wheelspeedPrev); wheelspeedPrev = [0 ;0 ;0 ;0]; end
persistent inertia; if isempty(inertia); inertia = car.tireInertia; end
if isempty(v); v =0;end
wheelspeed = sensors.wheelspeed;
alpha = (wheelspeed - wheelspeedPrev)/car.dt;

%wheelTorque = car.gearRatio*sensors.torque -(car.motor.Inertia*car.gearRatio^2 - car.tireInertia)*alpha;
%to be used if only motor torque is known (real scenario)

%Fxi_est = (wheelTorque - alpha*inertia)/car.tireRadius;
Fxi_est = (sensors.torque - alpha*inertia)/car.tireRadius;
%Fxi_est = (sensors.torque)/car.tireRadius;

Fx_tot = sensors.ax*car.mass + 0.5*car.rhoAir*v^2*car.Cd*car.AFront;
Fxi = Fxi_est;




wheelspeedPrev=wheelspeed;
inertiaOut = inertia;

== matlab function Torque_Vectoring_Controller_dSpace_RTI1401/Controls/Vehicle Estimated Parameters/Velocity Estimator/Velocity Estimator 1 ==
  data: sensors input; v1 output; settings input; car parameter
function v1  = Velocity_Estimator1(sensors, settings,  car)

%x-axis forward
%y-axis left
%z-axis upwards

tw_dist = [car.tw/2; -car.tw/2; car.tw/2; -car.tw/2];    

omegaR = max(sensors.wheelspeed*car.tireRadius,0);

persistent v_last; if (isempty(v_last)); v_last = 0; end

%estimate vi
vi = omegaR - tw_dist.*sensors.yawRate;
vi = vi .* cos(sensors.wheelAngles); 

%Front/rear best speed estimation
ax=sensors.ax;
limitax = 10;

vl = vi([1 3]);
vr = vi([2 4]);

if (ax > limitax)
   vsetl=min(vl);
   vsetr=min(vr);
elseif (ax < -limitax)
   vsetl=max(vl);
   vsetr=max(vr);
else
   vsetl=(min(vl)*(limitax + ax) + max(vl)*(limitax - ax))/(2*limitax);
   vsetr=(min(vr)*(limitax + ax) + max(vr)*(limitax - ax))/(2*limitax);
end
    
%left/right best speed estimation
ay=sensors.ay;
limitay = 20;

if (ay > limitay)
   v_est = vsetr;
elseif (ay < -limitay)
   v_est = vsetl;
else
   v_est = (vsetr*(ay + limitay) + vsetl*(limitay-ay))/(2*limitay);
end

v1=v_est;
%v=mean(omegaR);

== matlab function Torque_Vectoring_Controller_dSpace_RTI1401/Controls/Control Systems/Distributor/MATLAB Function ==
  data: sensors input; torqueDistribution output; settings input; estimPar input; car parameter; variables input; Mz input; slipSet output; Fdes output; sumFx output; Fxmax output; Fxmaxsum output; Fx output; Fdes input
function [torqueDistribution, slipSet,Fdes,sumFx,Fxmax,Fxmaxsum, Fx]= TorqueDistributor(sensors,settings, estimPar, car, variables, Mz, Fdes)
%,Fdes,sumFx,Fxmax,Fxmaxsum

torqueDistribution = [0;0;0;0];
slipSet = [0;0;0;0];


sumFx=0;
Fxmax=[0;0;0;0];
Fxmaxsum=0;
Fx=[0;0;0;0];
if settings.torqueMode == 1
    
    dT =  0.25*Mz/(car.tw*0.5)*car.tireRadius;
    torqueDistribution = car.motor.Tmax*variables.TD_percentage*sensors.throttle;
    torqueDistribution = torqueDistribution + [-1; 1; -1; 1]*dT;
    
    for i=1:4
        if torqueDistribution(i) > 0
            slipSet(i) = car.TC.slipSetAcc;
        else
            slipSet(i) = car.TC.slipSetBrake;
        end
    end
    
    
end



%Test torque mode: only Fx, no steeringAngle

if settings.torqueMode == 2
    

    
    Fxmax = [0;0;0;0];
    %minForce = 2*car.Cd*car.AFront*0.5*car.rhoAir*estimPar.v*estimPar.v*0.25; %2* of niet? en met Cd?
    minForce = 0;
    %FyReduceFactor = 0.1;
    %Fxmax = (max((estimPar.mu .* estimPar.Fzi).^2-FyReduceFactor*estimPar.Fyi.^2,0).^0.5); %Kamm's circle
    
    
    
    Fxmax = estimPar.mu.*estimPar.Fzi;
    
    Fxmax = max(Fxmax,minForce);
    
    FxmaxMax = car.gearRatio*car.motor.Tmax/car.tireRadius; %make sure the max torque of the motor isn't surpassed
    checkFxmax = find((Fxmax > FxmaxMax)==1);
    Fxmax(checkFxmax)=FxmaxMax(checkFxmax);
    
    if settings.unlimitedFx == 1  %Surpass the tire grip limits in case if the driver feels to restricted with this.
        Fxmax = FxmaxMax;
    end
    
    Fxmaxsum = sum(Fxmax);
    Fxmin = -Fxmax;
    
    Fx = [0;0;0;0];
    
    
    Fx = Distributor(settings, car, Mz, Fdes, Fxmax, Fxmin);
    
    torqueDistribution = car.tireRadius*Fx; %torque of motor, NOT of wheels (as IPG expects this as input)
    
    for i=1:4
        if torqueDistribution(i) > 0
            slipSet(i) = car.TC.slipSetAcc;
        else
            slipSet(i) = car.TC.slipSetBrake;
        end
    end
    
    sumFx = sum(Fx);
end


end

== matlab function Torque_Vectoring_Controller_dSpace_RTI1401/Controls/Bypass/MATLAB Function ==
  data: settings input; torqueBypass output; sensors input; rpmBypass output; car parameter
function [torqueBypass,rpmBypass]= fcn(settings, sensors, car)
PmaxTyre = car.Pmax_bypass*0.25;
rad2rpm = 30/pi;


safetyFactor = 0.5;
torqueBypass = car.motor.Tmax*safetyFactor*car.gearRatio*sensors.throttle;

if sensors.throttle > 0
    rpmBypass = car.motor.rpmMax;
else
    rpmBypass = [0;0;0;0];
end

%% Power limiter
limit = PmaxTyre./max(sensors.wheelspeed,1);
torqueBypass = max(min(torqueBypass,limit),-limit);

== matlab function Torque_Vectoring_Controller_dSpace_RTI1401/Controls/Vehicle Estimated Parameters/Velocity Estimator/Velocity_Estimator4 ==
  data: sensors input; v4 output; settings input; Fyi input; car parameter
function v4  = Velocity_Estimator4(sensors, settings,Fyi,  car)

% Based on "Vehicle velocity estimation using effective inertia for an in-wheel
% elecric vehicle"

SumLongitudinalForce=0;




persistent wheelspeedPrev; if isempty(wheelspeedPrev); wheelspeedPrev = [0 ;0 ;0 ;0]; end
persistent vPrev; if isempty(vPrev); vPrev = 0; end
persistent v4dot; if isempty(v4dot); v4dot = 0; end
wheelspeed = sensors.wheelspeed;

alpha = (wheelspeed - wheelspeedPrev)/car.dt;

Fresist = 0.5*car.Cd*car.AFront*car.rhoAir*vPrev^2; % moet nauwkeuriger


SumLongitudinalForce = sum(sensors.torque-alpha*car.tireInertia)/car.tireRadius...
    - Fresist;
Meff = SumLongitudinalForce/sensors.ax; %effective inertia / virtual mass


v4dot = (-(Fyi(1)*sin(sensors.wheelAngles(1))+Fyi(2)*sin(sensors.wheelAngles(2)))...
    + SumLongitudinalForce) / Meff;




v4 = vPrev + v4dot*car.dt;

vPrev = v4;




end

== matlab function Torque_Vectoring_Controller_dSpace_RTI1401/Controls/Vehicle Estimated Parameters/Fy Estimator  ==
  data: sensors input; Fyi output; settings input; Fzi input; Fxi input; car parameter; optPar parameter
function Fyi = Fy_Estimator(sensors, settings, Fzi, Fxi, car,optPar)

Fyi=[0;0;0;0];
persistent yawRatePrev; if isempty(yawRatePrev); yawRatePrev = sensors.yawRate; end
persistent M_Fx; if isempty(M_Fx); M_Fx = 0; end
persistent M_Fy; if isempty(M_Fy); M_Fy = 0; end
persistent FyRear; if isempty(FyRear); FyRear = 0; end
persistent FzRatioFront; if isempty(FzRatioFront);FzRatioFront = 0; end
persistent FzRatioRear; if isempty(FzRatioRear); FzRatioRear = 0; end
persistent FyFront; if isempty(FyFront); FyFront = 0; end
persistent Fy_FL; if isempty(Fy_FL); Fy_FL = 0; end

yawAcc = (sensors.yawRate - yawRatePrev) * car.fECU;

wheelAngle = (sensors.wheelAngles(1)+sensors.wheelAngles(2))/2;

%Calculate contributions to the moment from lateral forces through the
%total yaw moment and moment of the longitudinal forces.
M_YawTot = car.yawInertia*yawAcc;
M_Fx = (car.tw/2)*cos(wheelAngle)*(Fxi(1)-Fxi(2))...
    +car.lf*sin(wheelAngle)*(Fxi(1)+Fxi(2))...
    +(car.tw/2)*(Fxi(3)-Fxi(4));
M_Fy = M_YawTot - M_Fx;

%Distribution of lateral force on front and rear axle
%NOTE %sin(steerinAngle) deel wordt momenteel verwaarloosd
%     %--> FyFR - FyFL =~ 0
Fy = car.mass*sensors.ay;
FyRear = (cos(wheelAngle)*car.lf*Fy - M_Fy)/...
    (cos(wheelAngle)*car.lf+car.lr);
FyFront = Fy - FyRear;

%Distribution of lateral force on left and right tire by using the normal
%force distribution.

%Use of a scale factor 

FzRatioFront = [Fzi(1); Fzi(2)]./sum(Fzi(1:2));
FzRatioRear = [Fzi(3); Fzi(4)]./sum(Fzi(3:4));



FyFrontDiff = (FzRatioFront(1) - FzRatioFront(2))*optPar.scaleFactorFy/2;
Fy_FL = FyFront/2 + FyFrontDiff* FyFront;
Fy_FR = FyFront/2 - FyFrontDiff* FyFront;
FyRearDiff = (FzRatioRear(1) - FzRatioRear(2))*optPar.scaleFactorFy/2;
Fy_RL = FyRear/2 + FyRearDiff* FyRear;
Fy_RR = FyRear/2 - FyRearDiff* FyRear;
    
Fyi=[Fy_FL;Fy_FR;Fy_RL;Fy_RR];

yawRatePrev=sensors.yawRate;

== matlab function Torque_Vectoring_Controller_dSpace_RTI1401/Controls/Vehicle Estimated Parameters/Aerodynamic forces ==
  data: sensors input; aero output Bus: aeroBus; settings input; v input; car parameter
function aero = aerodynamics(sensors, settings, v, car)

% === from dataCar.m ===
% car.Cl = 3.84;      %[-]   %Lift coefficient
% car.Cd = 1.44;      %[-]   %Drag coefficient
% car.AFront = 1.3;   %[m^2] %Frontal area
% car.rhoAir = 1.225; %[kg/m^3] %air density

aero.FD = 0.5*car.Cd*car.AFront*car.rhoAir*v^2; %drag force, pointing rearward [N]
aero.FL = 0.5*car.Cl*car.AFront*car.rhoAir*v^2; %lift force, pointing upward [N]
aero.lever_FD = [-0.1;0.1]; %distance from the COG to the point of application of the drag [m]
aero.lever_FL = [-0.1;0.1]; %distance from the COG to the point of application of the lift [m]

== matlab function Torque_Vectoring_Controller_dSpace_RTI1401/Controls/Vehicle Estimated Parameters/Estim Par ==
  data: v input; estimPar output Bus: estimParBus; Fzi input; Fxi input; Fyi input; rref input; mu input; slip input; eff input
function estimPar = fcn(v,Fzi,Fxi,Fyi,rref,mu,slip,eff)

estimPar.v=v;
estimPar.Fzi=Fzi;
estimPar.Fxi=Fxi;
estimPar.Fyi=Fyi;
estimPar.rref=rref;
estimPar.mu=mu;
estimPar.slip=slip;
estimPar.eff=eff;
